simulink model "simulate_DSBTC_MATLAB"  (R2021a)
settings: Solver=VariableStepAuto  StartTime=0.0  StopTime=2  RelTol=1e-3
InitFcn:
  | fs = 4000;
  | frameSize = 512;
libraries: dspsrcs4 x1
settings Model: Creator=Byung-Jun Jang  LastModifiedBy=user
settings SolverCC: AlgebraicLoopSolver=TrustRegion
settings DataIOCC: ReturnWorkspaceOutputs=off
settings DebuggingCC: SFMachineParentedDataDiag=warning  ArithmeticOperatorsInVariantConditions=warning
settings SFSimCC: SimUseLocalCustomCode=off  CustomCodeUndefinedFunction=UseInterfaceOnly
settings RTWCC: RTWUseLocalCustomCode=off
settings CodeAppCC: StateflowObjectComments=on
settings SimscapeCC: SimscapeNormalizeSystem=off

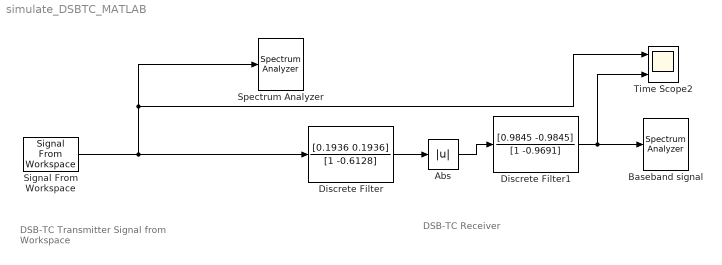
== system simulate_DSBTC_MATLAB ==
  note: DSB-TC Transmitter
      | Signal from Workspace
  note: DSB-TC Receiver
  Abs : Abs
  Baseband signal : SpectrumAnalyzer
  Discrete Filter : DiscreteFilter  Numerator=[0.1936 0.1936]  Denominator=[1 -0.6128]  InputProcessing=Columns as channels (frame based)  FilterStructure=Direct form II transposed  a0EqualsOne=on
  Discrete Filter1 : DiscreteFilter  Numerator=[0.9845 -0.9845]  Denominator=[1 -0.9691]  InputProcessing=Columns as channels (frame based)  FilterStructure=Direct form II transposed  a0EqualsOne=on
  Signal From Workspace : dspsrcs4/Signal From Workspace  X=r  Ts=1/fs  nsamps=frameSize  OutputAfterFinalValue=Cyclic repetition  ignoreOrWarnInputAndFrameLengths=off  OutputFrames=off
  Spectrum Analyzer : SpectrumAnalyzer
  Time Scope2 : Scope  NumInputPorts=2
  wires:
  Signal From Workspace/1 -> Spectrum Analyzer/1, Time Scope2/1, Discrete Filter/1
  Abs/1 -> Discrete Filter1/1
  Discrete Filter1/1 -> Time Scope2/2, Baseband signal/1
  Discrete Filter/1 -> Abs/1
